simulink model "Ejercicio_3_DB"  (R2023a)
settings: Solver=VariableStepAuto  StartTime=0.0  StopTime=10.0  RelTol=1e-3
values from neighbouring files (symbols this model uses):
  A = [0 1 0 0; 0 0 -m*g/M 0; 0 0 0 1; 0 0 g*(M+m)/(l*M) 0]    [Ejercicio_1.m]    (also in Ejercicio_3.m)
  B = [0; 1/M ; 0; -1/(l*M)]    [Ejercicio_1.m]    (also in Ejercicio_3.m)
  g0 = utilsMati.realim_VE.factorEscala(A,B,C,K)    [Ejercicio_3.m]
  K = acker(A,B,PLC)    [Ejercicio_3.m]
settings Model: Creator=Mati  LastModifiedBy=Mati

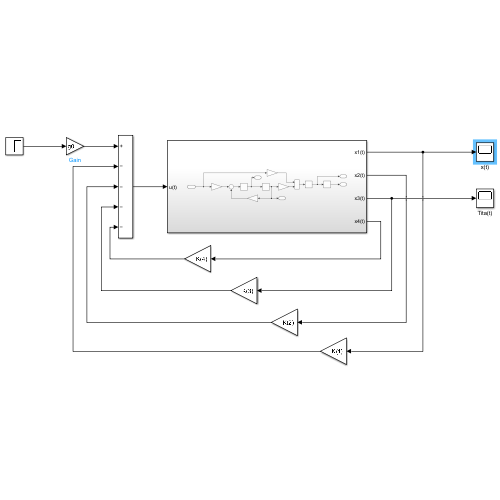
[thumbnail: Simulink's stored preview of the top-level diagram]
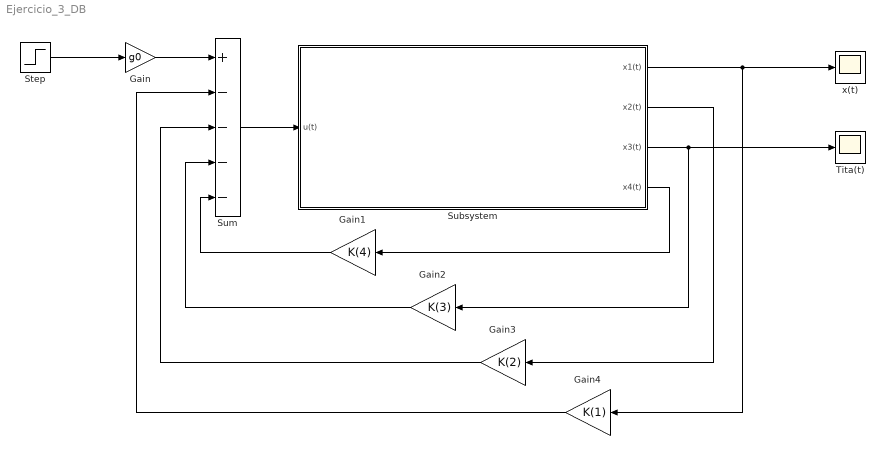
== system Ejercicio_3_DB ==
  Gain : Gain  Gain=g0
  Gain1 : Gain  Gain=K(4)
  Gain2 : Gain  Gain=K(3)
  Gain3 : Gain  Gain=K(2)
  Gain4 : Gain  Gain=K(1)
  Step : Step  SampleTime=0
  Subsystem : Subsystem
  Sum : Sum  Inputs=+----
  Tita(t) : Scope
  x(t) : Scope
  wires:
  Gain/1 -> Sum/1
  Step/1 -> Gain/1
  Sum/1 -> Subsystem/1(u(t))
  Gain1/1 -> Sum/5
  Subsystem/4(x4(t)) -> Gain1/1
  Gain2/1 -> Sum/4
  Subsystem/3(x3(t)) -> Tita(t)/1, Gain2/1
  Gain3/1 -> Sum/3
  Gain4/1 -> Sum/2
  Subsystem/2(x2(t)) -> Gain3/1
  Subsystem/1(x1(t)) -> x(t)/1, Gain4/1

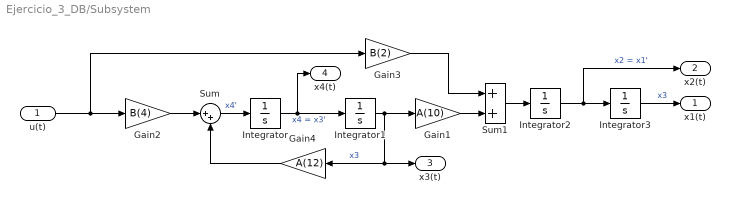
== system Ejercicio_3_DB/Subsystem ==
  u(t) : Inport
  Gain1 : Gain  Gain=A(10)
  Gain2 : Gain  Gain=B(4)
  Gain3 : Gain  Gain=B(2)
  Gain4 : Gain  Gain=A(12)
  Integrator{,1..3} (4 alike) : Integrator
  Sum : Sum  Inputs=|++
  Sum1 : Sum
  x1(t) : Outport
  x2(t) : Outport  Port=2
  x3(t) : Outport  Port=3
  x4(t) : Outport  Port=4
  wires:
  Gain2/1 -> Sum/1
  Sum/1 -> Integrator/1  "x4'"
  Integrator/1 -> Integrator1/1, x4(t)/1  "x4 = x3'"
  Integrator1/1 -> Gain1/1, Gain4/1, x3(t)/1  "x3"
  u(t)/1 -> Gain3/1, Gain2/1
  Gain1/1 -> Sum1/2
  Gain3/1 -> Sum1/1
  Gain4/1 -> Sum/2
  Sum1/1 -> Integrator2/1
  Integrator2/1 -> x2(t)/1, Integrator3/1  "x2 = x1'"
  Integrator3/1 -> x1(t)/1  "x3"
